simulink model "Mech_vent"  (Simulink 6.4)
settings: Solver=ode45  StartTime=0.0  StopTime=10.0  RelTol=1e-3
values from neighbouring files (symbols this model uses):
  Mech_Vent_pressure = 17    [Mech_vent_test.m]
  t_Mech_Vent_duration = 0    [Mech_vent_test.m]
  t_Mech_Vent_start = 0    [Mech_vent_test.m]
undefined symbols (not defined in the file or in its folder): CPAP_pressure, t_CPAP_duration, t_CPAP_start
settings Model: LastModifiedBy=CLM

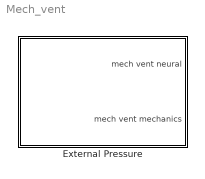
== system Mech_vent ==
  External Pressure : Subsystem
      mask Display: image(imread('CPAP2.bmp'))

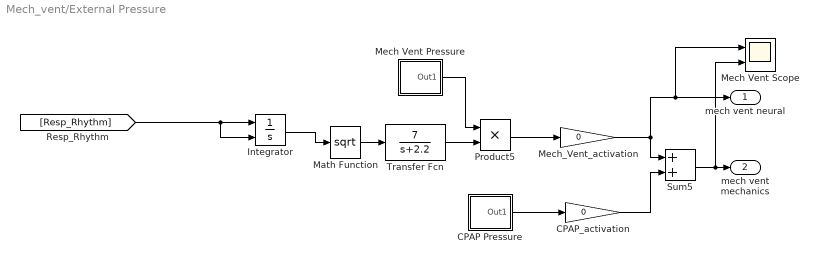
== system Mech_vent/External Pressure ==
  CPAP Pressure : Subsystem  mask{begin_time=t_CPAP_start, end_time=t_CPAP_start+t_CPAP_duration, init_value=0, final_value=CPAP_pressure}
      mask prompts: begin_time "pulse begin"; end_time "pulse end"; init_value "initial value"; final_value "final value"
      mask Display: disp('pulse')
  CPAP_activation : Gain  Gain=0  SaturateOnIntegerOverflow=on
  Integrator : Integrator  ExternalReset=falling
  Math Function : Math  Operator=sqrt  SaturateOnIntegerOverflow=on
  Mech Vent Pressure : Subsystem  mask{begin_time=t_Mech_Vent_start, end_time=t_Mech_Vent_start+t_Mech_Vent_duration, init_value=0, final_value=Mech_Vent_pressure}
      mask prompts: begin_time "pulse begin"; end_time "pulse end"; init_value "initial value"; final_value "final value"
      mask Display: disp('pulse')
  Mech Vent Scope : Scope  NumInputPorts=2
      settings: TimeRange=100  YMin=0~0  YMax=75~75  SaveName=ScopeData14  MaxDataPoints=50
  Mech_Vent_activation : Gain  Gain=0  SaturateOnIntegerOverflow=on
  Product5 : Product  SaturateOnIntegerOverflow=on  InputSameDT=on
  Sum5 : Sum  SaturateOnIntegerOverflow=on  InputSameDT=on
  Transfer Fcn : TransferFcn  Numerator=[7]  Denominator=[1 2.2]
  mech vent neural : Outport
  mech vent mechanics : Outport  Port=2
  wires:
  Sum5/1 -> mech vent mechanics/1, Mech Vent Scope/2
  [Resp_Rhythm] -> Integrator/1, Integrator/2
  Integrator/1 -> Math Function/1
  Math Function/1 -> Transfer Fcn/1
  Transfer Fcn/1 -> Product5/2
  Product5/1 -> Mech_Vent_activation/1
  CPAP Pressure/1(Out1) -> CPAP_activation/1
  CPAP_activation/1 -> Sum5/2
  Mech_Vent_activation/1 -> Sum5/1, mech vent neural/1, Mech Vent Scope/1
  Mech Vent Pressure/1(Out1) -> Product5/1

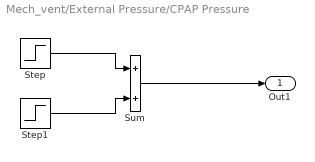
== system Mech_vent/External Pressure/CPAP Pressure ==
  Step : Step  Time=begin_time  Before=init_value  After=final_value  SampleTime=0
  Step1 : Step  Time=end_time  After=init_value-final_value  SampleTime=0
  Sum : Sum  Inputs=|++  SaturateOnIntegerOverflow=on  InputSameDT=on
  Out1 : Outport
  wires:
  Sum/1 -> Out1/1
  Step1/1 -> Sum/2
  Step/1 -> Sum/1

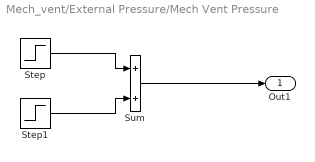
== system Mech_vent/External Pressure/Mech Vent Pressure ==
  Step : Step  Time=begin_time  Before=init_value  After=final_value  SampleTime=0
  Step1 : Step  Time=end_time  After=init_value-final_value  SampleTime=0
  Sum : Sum  Inputs=|++  SaturateOnIntegerOverflow=on  InputSameDT=on
  Out1 : Outport
  wires:
  Step/1 -> Sum/1
  Step1/1 -> Sum/2
  Sum/1 -> Out1/1
